simulink model "Child_Model"  (R2014a)
settings: Solver=FixedStepDiscrete  StartTime=0.0  StopTime=10.0  FixedStep=1/400  RelTol=1e-3
libraries: simulink x2
settings Model: Creator=darenlee  LastModifiedBy=darenlee
settings SolverCC: PositivePriorityOrder=on
settings OptimizationCC: OptimizeModelRefInitCode=on  LifeSpan=1  MaxStackSize=64
settings HardwareCC: ProdLargestAtomicInteger=Long  ProdLargestAtomicFloat=Double  ProdEndianess=LittleEndian  ProdHWDeviceType=ARM Compatible->ARM Cortex
settings RTWCC: SystemTargetFile=ert.tlc  TLCOptions=-aInlineSetEventsForThisBaseRateFcn=TLC_FALSE -aSuppressMultiTaskScheduler=TLC_FALSE  TemplateMakefile=ert_default_tmf  Description=Embedded Coder  GenerateReport=on  ProcessScript=ert_make_rtw_hook  Toolchain=Code Sourcery  IncludeHyperlinkInReport=on  LaunchReport=on  CodeExecutionProfiling=on  CodeProfilingSaveOptions=AllData  CodeProfilingInstrumentation=on  GenerateTraceInfo=on  GenerateTraceReport=on  GenerateTraceReportSl=on  GenerateTraceReportSf=on  GenerateTraceReportEml=on  GenerateCodeMetricsReport=on  GenerateCodeReplacementReport=on
settings CodeAppCC: IgnoreCustomStorageClasses=off
settings ERTTargetCC: ParMdlRefBuildCompliant=on  CompOptLevelCompliant=on  ConcurrentExecutionCompliant=on  ERTFirstTimeCompliant=on  ModelStepFunctionPrototypeControlCompliant=on  CPPClassGenCompliant=on  InlinedParameterPlacement=Hierarchical

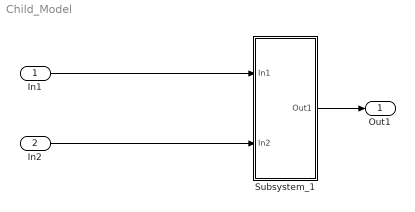
== system Child_Model ==
  In1 : Inport
  In2 : Inport  Port=2
  Subsystem_1 : Subsystem  TreatAsAtomicUnit=on
  Out1 : Outport
  wires:
  In1/1 -> Subsystem_1/1(In1)
  In2/1 -> Subsystem_1/2(In2)
  Subsystem_1/1(Out1) -> Out1/1

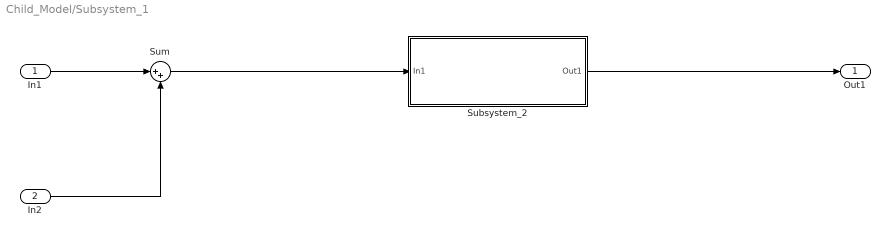
== system Child_Model/Subsystem_1 ==
  In1 : Inport
  In2 : Inport  Port=2
  Subsystem_2 : Subsystem  TreatAsAtomicUnit=on
  Sum : Sum  Inputs=|++
  Out1 : Outport
  wires:
  In1/1 -> Sum/1
  In2/1 -> Sum/2
  Sum/1 -> Subsystem_2/1(In1)
  Subsystem_2/1(Out1) -> Out1/1

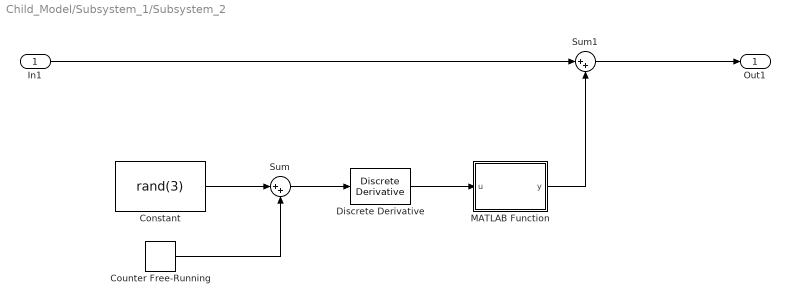
== system Child_Model/Subsystem_1/Subsystem_2 ==
  In1 : Inport
  Constant : Constant  Value=rand(3)
  Counter Free-Running : simulink/Sources/Counter Free-Running  NumBits=16  tsamp=-1
  Discrete Derivative : simulink/Discrete/Discrete Derivative  gainval=1.0  ICPrevScaledInput=0.0  InputProcessing=Inherited  OutMin=[]  OutMax=[]  OutDataType=fixdt(1, 16)  OutScaling=2^-10  DoSatur=off
  MATLAB Function : MATLAB Function  TreatAsAtomicUnit=on
  Sum : Sum  Inputs=|++
  Sum1 : Sum  Inputs=|++
  Out1 : Outport
  wires:
  Discrete Derivative/1 -> MATLAB Function/1(u)
  MATLAB Function/1(y) -> Sum1/2
  In1/1 -> Sum1/1
  Sum1/1 -> Out1/1
  Constant/1 -> Sum/1
  Sum/1 -> Discrete Derivative/1
  Counter Free-Running/1 -> Sum/2

== matlab function Child_Model/Subsystem_1/Subsystem_2/MATLAB Function ==
  data: u input; y output
function y = fcn(u)
%#codegen

y = u(3,3);
